simulink model "pid"  (R2022b)
settings: Solver=VariableStepAuto  StartTime=0.0  StopTime=10.0  RelTol=1e-3
settings Model: Creator=ardac  LastModifiedBy=ardac

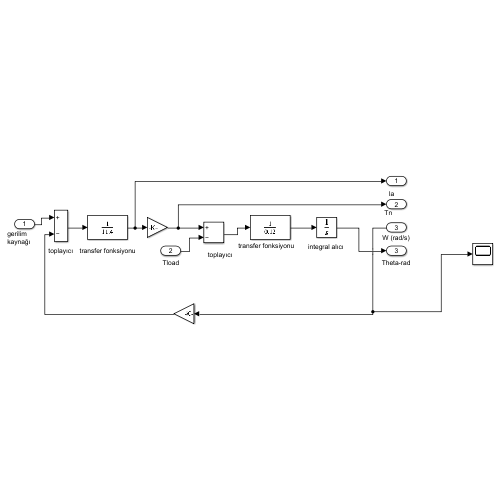
[thumbnail: Simulink's stored preview of the top-level diagram]
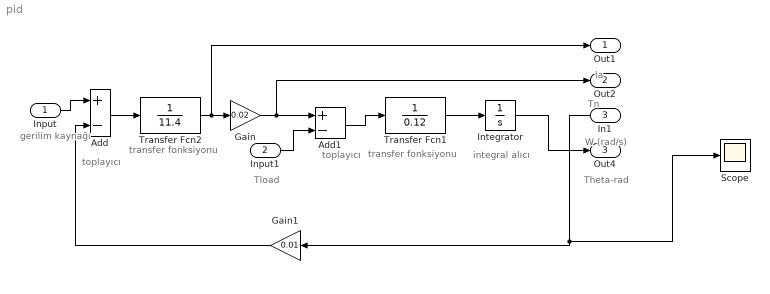
== system pid ==
  note: Theta-rad
  note: W (rad/s)
  note: Tn
  note: la
  note: integral alıcı
  note: transfer fonksiyonu
  note: toplayıcı
  note: gerilim kaynağı
  note: transfer fonksiyonu
  note: Tload
  note: toplayıcı
  Input : Inport
  Input1 : Inport  Port=2
  In1 : Inport  Port=3
  Add : Sum  Inputs=+-
  Add1 : Sum  Inputs=+-
  Gain : Gain  Gain=0.02
  Gain1 : Gain  Gain=0.01
  Integrator : Integrator
  Scope : Scope
  Transfer Fcn1 : TransferFcn  Denominator=0.12
  Transfer Fcn2 : TransferFcn  Denominator=11.4
  Out1 : Outport
  Out2 : Outport  Port=2
  Out4 : Outport  Port=3
  wires:
  Input/1 -> Add/1
  Add/1 -> Transfer Fcn2/1
  Transfer Fcn2/1 -> Out1/1, Gain/1
  Input1/1 -> Add1/2
  Gain/1 -> Out2/1, Add1/1
  Transfer Fcn1/1 -> Integrator/1
  Integrator/1 -> Out4/1
  Add1/1 -> Transfer Fcn1/1
  Gain1/1 -> Add/2
  In1/1 -> Scope/1, Gain1/1
